simulink model "atrialfib"  (R2016b)
settings: Solver=ode45  StartTime=0.0  StopTime=1.6  FixedStep=1e-4  RelTol=1e-12  EnableMultiTasking=on
settings Model: Creator=amal029_old  LastModifiedBy=amal029_old
settings SolverCC: ZeroCrossAlgorithm=Adaptive  AutoInsertRateTranBlk=on
settings DataIOCC: LimitDataPoints=on
settings OptimizationCC: LifeSpan=inf
settings DebuggingCC: AllowSymbolicDim=off  SFUnexpectedBacktrackingDiag=warning  SFNoUnconditionalDefaultTransitionDiag=warning  SFExecutionAtInitializationDiag=none
settings GRTTargetCC: TargetLangStandard=C89/C90 (ANSI)
settings ConfigComp: CovMetricSettings=dw  CovHtmlReporting=on  CovSaveCumulativeToWorkspaceVar=on  CovSaveSingleToWorkspaceVar=on  CovShowResultsExplorer=off  CovExternalEMLEnable=off

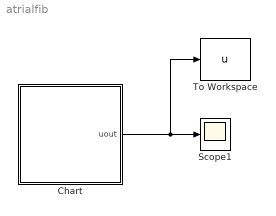
== system atrialfib ==
  Chart : Stateflow chart  TreatAsAtomicUnit=on
  Scope1 : Scope
  To Workspace : ToWorkspace  VariableName=u  SampleTime=-1
      settings: Save2DSignal=2-D array (concatenate along first dimension)
  wires:
  Chart/1(uout) -> To Workspace/1, Scope1/1

== stateflow chart atrialfib/Chart ==
  settings: updateMethod=CONTINUOUS
  state State2
    du:
    tau_dot = 1.0;
    u_dot=((stim - jfi2) - ((u/EPI_TO2) + jsi2));
    w_dot=(((0.94-w)/(EPI_TW1M + (EPI_TW2M - EPI_TW1M) * (1.0 / (1+exp(-2*EPI_KWM*(u - EPI_UWM)))))));
    v_dot=((-v/EPI_TV2M));
    s_dot=((((1/(1+exp(-2 * EPI_KS * (u - EPI_US)))) - s)/EPI_TS1));
    uout=u;
  state State3
    du:
    tau_dot=1.0;
    u_dot=((stim - jfi3) - ((1.0/(EPI_TSO1+((EPI_TSO2 - EPI_TSO1) * (1/(1+exp(-2 * EPI_KSO * (u - EPI_USO))))))) + (0 - (w * s)/EPI_TSI)));
    w_dot=((-w/EPI_TWP));
    v_dot=((-v/EPI_TV2M));
    s_dot=((((1/(1+exp(-2 * EPI_KS * (u - EPI_US)))) - s)/EPI_TS2)); uout=u;
  state State4
    du:
    tau_dot=1.0;
    u_dot=((stim - (0 - v * (u - EPI_THV) * (EPI_UU - u)/EPI_TFI)) - ((1.0 / (EPI_TSO1+((EPI_TSO2 - EPI_TSO1) * (1/(1+exp(-2*EPI_KSO * (u - EPI_USO))))))) + (0 - (w * s)/EPI_TSI)));
    w_dot=((-w/EPI_TWP));
    v_dot=((-v/EPI_TVP));
    s_dot=((((1/(1+exp(-2 * EPI_KS * (u - EPI_US)))) - s)/EPI_TS2));
    uout=u;
  state State1
    du:
    tau_dot=1.0;
    u_dot = ((stim - jfi1) - ((u/EPI_TO1) + jsi1));
    w_dot=(((1.0 - (u / EPI_TWINF) - w) / (EPI_TW1M + (EPI_TW2M - EPI_TW1M) * (1.0 / (1 + exp(-2*EPI_KWM * (u - EPI_UWM)))))));
    v_dot=(((1.0 - v)/EPI_TV1M));
    s_dot=((((1/(1+ exp(-2 * EPI_KS * (u - EPI_US)))) - s)/EPI_TS1));
    uout=u;
  State2 -> State3 : [u >= 0.013]
  State1 -> State2 : [u >= 0.006]
  State3 -> State4 : [u >= 0.3]
  (default) -> State1 : {u=0; v=1.0; s=0; w=1.0; tau=0; uout=u;}
  State4 -> State4 : [u >= 2.0]
  data: EPI_TVP constant double size=1 =1.4506; EPI_TV1M constant double size=1 =60.0; EPI_TV2M constant double size=1 =1150.0; EPI_TWP constant double size=1 =200.0; EPI_TW1M constant double size=1 =60.0; EPI_TW2M constant double size=1 =15.0; EPI_TS1 constant double size=1 =2.7342; EPI_TS2 constant double size=1 =16.0; EPI_TFI constant double size=1 =0.11; EPI_TO2 constant double size=1 =6; EPI_TSO1 constant double size=1 =30.0181; EPI_TSO2 constant double size=1 =0.9957; EPI_TSI constant double size=1 =1.8875; EPI_TWINF constant double size=1 =0.07; EPI_THV constant double size=1 =0.3; EPI_KWM constant double size=1 =65.0; EPI_KS constant double size=1 =2.0994; EPI_KSO constant double size=1 =2.0458; EPI_UWM constant double size=1 =0.03; EPI_US constant double size=1 =0.9087; EPI_UU constant double size=1 =1.55; EPI_USO constant double size=1 =0.65; jfi1 constant double size=1 =0.0; jsi1 constant double size=1 =0.0; jfi2 constant double size=1 =0.0; jsi2 constant double size=1 =0.0; jfi3 constant double size=1 =0.0; stim constant double size=1 =1.0; s local; tau local; u local; v local; w local; EPI_TO1 constant double size=1 =0.007; uout output
  data s settings: updateMethod=SF_CONTINUOUS_TIME_DATA
  data tau settings: updateMethod=SF_CONTINUOUS_TIME_DATA
  data u settings: updateMethod=SF_CONTINUOUS_TIME_DATA
  data v settings: updateMethod=SF_CONTINUOUS_TIME_DATA
  data w settings: updateMethod=SF_CONTINUOUS_TIME_DATA
